simulink model "WindT_Control"  (R2026a)
settings: Solver=VariableStepAuto  StopTime=t(end)
InitFcn:
  | wtModelFile = get_param(bdroot, 'FileName'); wtProjectRoot = fileparts(fileparts(wtModelFile)); wtScriptsDir = fullfile(wtProjectRoot, 'scripts'); addpath(wtScriptsDir); init_wt(get_wind_case(), false);
model workspace (MAT data in the model file):
  surfaceBlockParameters = Simulink.LookupTable
  surfaceBlockParameters.Table = Simulink.lookuptable.Table
  surfaceBlockParameters.Table.Value = [0.000629396007942 0.006627327118 0.0623376026933 0.200719842793 0.356874891063 0.394066762825 0.350958924947 0.335467287882 0.311487736698 0.227563659042 0.0973704524374 0.0013612480249 ... (121 elements, 11x11)]
  surfaceBlockParameters.Table.Dimensions = [11 11]
  surfaceBlockParameters.Table.DataType = 'auto'
  surfaceBlockParameters.Table.FieldName = 'Table_Cp_'
  surfaceBlockParameters.Breakpoints(1) = Simulink.lookuptable.Breakpoint
  surfaceBlockParameters.Breakpoints(1).Value = [0.54 2.14 3.74 5.34 6.94 8.54 10.14 11.74 13.34 14.94 16.54]
  surfaceBlockParameters.Breakpoints(1).TunableSizeName = 'N1'
  surfaceBlockParameters.Breakpoints(1).TunableSizeValue = -1
  surfaceBlockParameters.Breakpoints(1).Dimensions = [1 11]
  surfaceBlockParameters.Breakpoints(1).DataType = 'auto'
  surfaceBlockParameters.Breakpoints(1).FieldName = 'BP1_Lambda'
  surfaceBlockParameters.Breakpoints(2) = Simulink.lookuptable.Breakpoint
  surfaceBlockParameters.Breakpoints(2).Value = [-8 -3.7 0.6 4.9 9.2 13.5 17.8 22.1 26.4 30.7 35]
  surfaceBlockParameters.Breakpoints(2).TunableSizeName = 'N2'
  surfaceBlockParameters.Breakpoints(2).TunableSizeValue = -1
  surfaceBlockParameters.Breakpoints(2).Dimensions = [1 11]
  surfaceBlockParameters.Breakpoints(2).DataType = 'auto'
  surfaceBlockParameters.Breakpoints(2).FieldName = 'BP2_Beta'
  surfaceBlockParameters.AllowMultipleInstancesOfTypeToHaveDifferentTableBreakpointSizes = 0
  surfaceBlockParameters.SupportTunableSize = 0
  surfaceBlockParameters.StructTypeInfo = Simulink.lookuptable.StructTypeInfo
  surfaceBlockParameters.StructTypeInfo.Name = 'surfaceBlockParameters_type'
  surfaceBlockParameters.StructTypeInfo.DataScope = 'Auto'
undefined symbols (not defined in the file): Beta_ott, C_rated, GBEff, GBRatio, GenEff, Jeq, Kreg2, Omega_0, Omega_ott_high, Omega_ott_low, R, rho
settings Model: Creator=39388  LastModifiedBy=notes

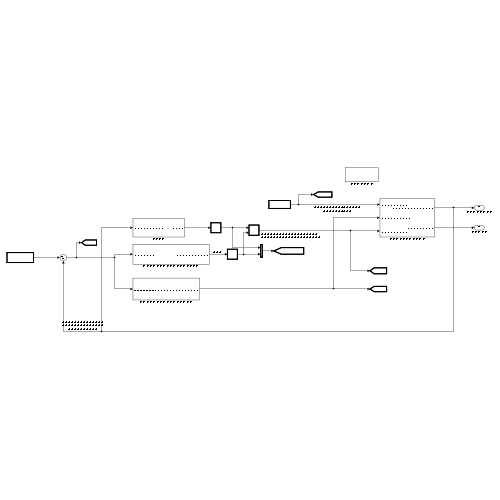
[thumbnail: Simulink's stored preview of the top-level diagram]
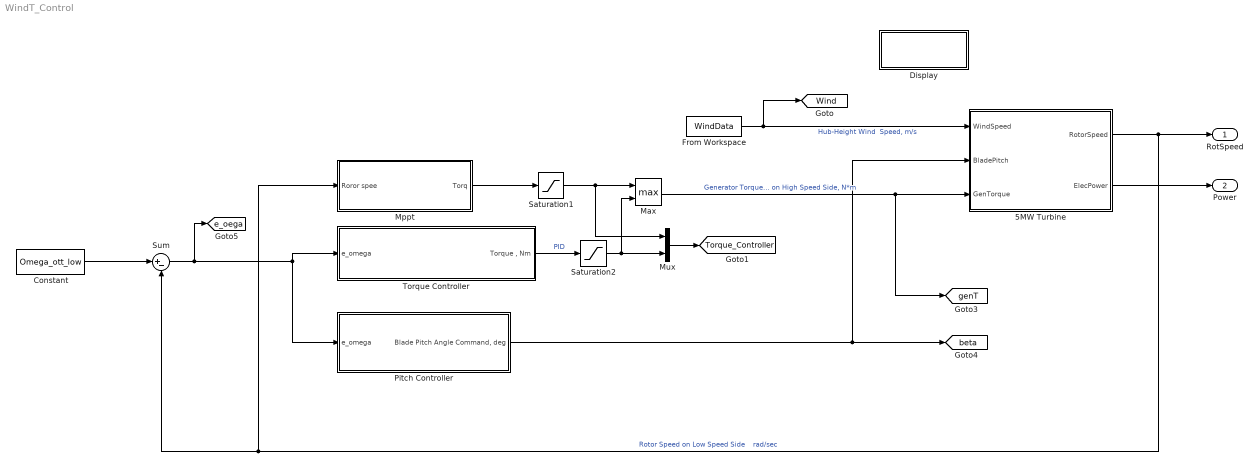
== system WindT_Control ==
  5MW Turbine : Subsystem
  Constant : Constant  Value=Omega_ott_low
  Display : Subsystem
  From Workspace : FromWorkspace  VariableName=WindData
  Max : MinMax  Function=max  Inputs=2
  Mppt : Subsystem
  Mux : Mux  Inputs=2
  Pitch Controller : Subsystem
  Saturation1 : Saturate  UpperLimit=Omega_ott_high^2*Kreg2  LowerLimit=0
  Saturation2 : Saturate  UpperLimit=C_rated/GBRatio  LowerLimit=0
  Sum : Sum  Inputs=|+-
  Torque Controller : Subsystem
  RotSpeed : Outport
  Power : Outport  Port=2
  tag scope: Torque_Controller=global, Wind=global, beta=global, e_oega=global, genT=global
  wires:
  5MW Turbine/2(ElecPower) -> Power/1
  From Workspace/1 -> [Wind], 5MW Turbine/1(WindSpeed)  "Hub-Height Wind  Speed, m/s"
  Pitch Controller/1("Blade Pitch Angle Command, deg") -> [beta], 5MW Turbine/2(BladePitch)
  Mux/1 -> [Torque_Controller]
  Constant/1 -> Sum/1
  Max/1 -> 5MW Turbine/3(GenTorque), [genT]  "Generator Torque on High Speed Side, N*m"
  Torque Controller/1("Torque , Nm") -> Saturation2/1  "PID"
  Mppt/1(Torq) -> Saturation1/1
  5MW Turbine/1("RotorSpeed ") -> RotSpeed/1, Mppt/1(Roror spee), Sum/2  "Rotor Speed on Low Speed Side    rad/sec"
  Sum/1 -> [e_oega], Torque Controller/1(e_omega), Pitch Controller/1(e_omega)
  Saturation1/1 -> Mux/1, Max/1
  Saturation2/1 -> Mux/2, Max/2

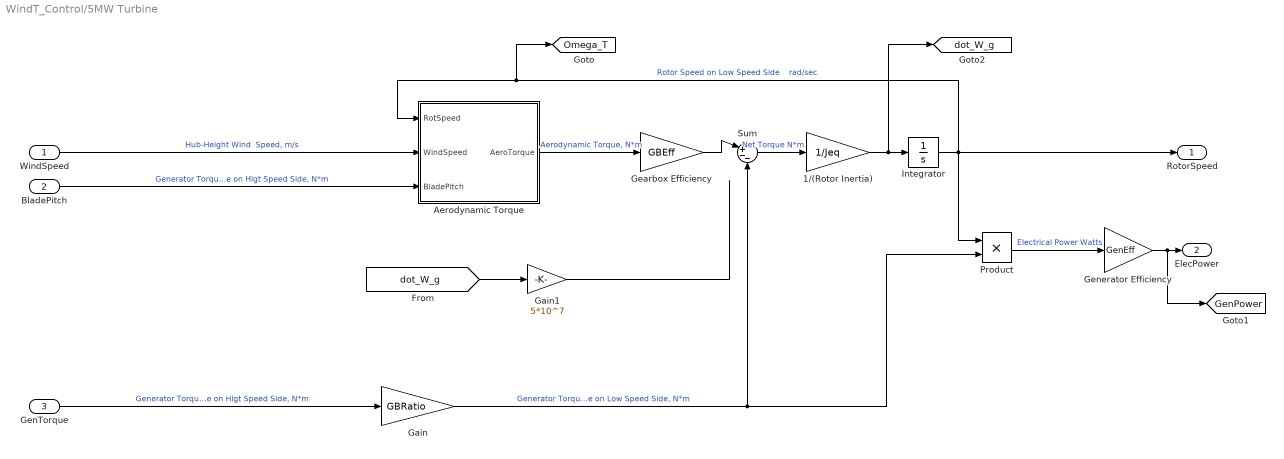
== system WindT_Control/5MW Turbine ==
  WindSpeed : Inport
  BladePitch : Inport  Port=2
  GenTorque : Inport  Port=3
  1/(Rotor Inertia) : Gain  Gain=1/Jeq
  Aerodynamic Torque : Subsystem
  Gain : Gain  Gain=GBRatio
  Gain1 : Gain  Gain=5*10^7
  Gearbox Efficiency : Gain  Gain=GBEff
  Generator Efficiency : Gain  Gain=GenEff
  Integrator : Integrator  InitialCondition=Omega_0
  Product : Product  Inputs=**
  Sum : Sum  Inputs=|+--
  "RotorSpeed " : Outport
  ElecPower : Outport  Port=2
  tag scope: GenPower=global, Omega_T=global, dot_W_g=global
  wires:
  Integrator/1 -> "RotorSpeed "/1, Product/1, [Omega_T], Aerodynamic Torque/1("RotSpeed ")  "Rotor Speed on Low Speed Side    rad/sec"
  Sum/1 -> 1/(Rotor Inertia)/1  "Net Torque N*m"
  Gearbox Efficiency/1 -> Sum/1
  Gain/1 -> Product/2, Sum/3  "Generator Torque on Low Speed Side, N*m"
  1/(Rotor Inertia)/1 -> [dot_W_g], Integrator/1
  WindSpeed/1 -> Aerodynamic Torque/2(WindSpeed)  "Hub-Height Wind  Speed, m/s"
  Aerodynamic Torque/1(AeroTorque) -> Gearbox Efficiency/1  "Aerodynamic Torque, N*m"
  Product/1 -> Generator Efficiency/1  "Electrical Power Watts"
  Generator Efficiency/1 -> [GenPower], ElecPower/1
  BladePitch/1 -> Aerodynamic Torque/3(BladePitch)  "Generator Torque on Higt Speed Side, N*m"
  GenTorque/1 -> Gain/1  "Generator Torque on Higt Speed Side, N*m"
  [dot_W_g] -> Gain1/1
  Gain1/1 -> ?

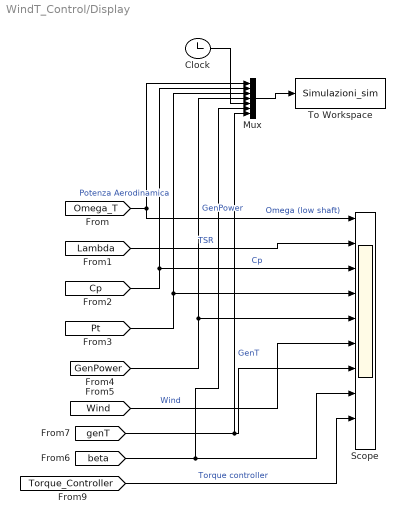
== system WindT_Control/Display ==
  Clock : Clock
  Mux : Mux  Inputs=7
  Scope : Scope  NumInputPorts=10
      settings: ActiveDisplayYMinimum=1.05767  ActiveDisplayYMaximum=1.34149
  To Workspace : ToWorkspace  VariableName=Simulazioni_sim  SampleTime=-1
  wires:
  [Omega_T] -> Mux/1, Scope/1  "Omega (low shaft)"
  [Pt] -> Mux/3, Scope/4  "Potenza Aerodinamica"
  [Lambda] -> Scope/2  "TSR"
  [Cp] -> Mux/2, Scope/3  "Cp"
  [GenPower] -> Mux/4, Scope/5  "GenPower"
  [Wind] -> Scope/6  "Wind"
  Mux/1 -> To Workspace/1
  Clock/1 -> Mux/5
  [beta] -> Mux/6, Scope/8
  [genT] -> Mux/7, Scope/7  "GenT"
  [Torque_Controller] -> Scope/9  "Torque controller"

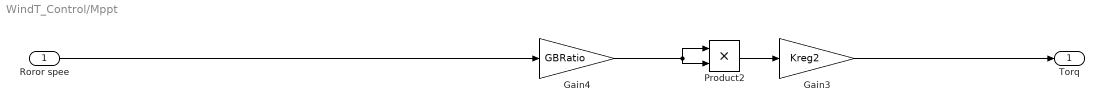
== system WindT_Control/Mppt ==
  Roror spee : Inport
  Gain3 : Gain  Gain=Kreg2
  Gain4 : Gain  Gain=GBRatio
  Product2 : Product
  Torq : Outport
  wires:
  Gain4/1 -> Product2/1, Product2/2
  Gain3/1 -> Torq/1
  Roror spee/1 -> Gain4/1
  Product2/1 -> Gain3/1

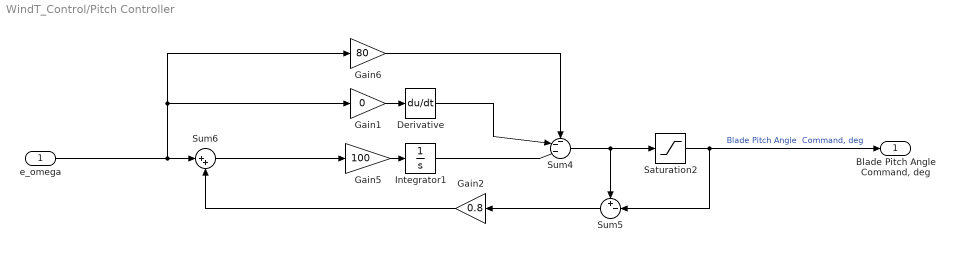
== system WindT_Control/Pitch Controller ==
  e_omega : Inport
  Derivative : Derivative
  Gain1 : Gain  Gain=0
  Gain2 : Gain  Gain=0.8
  Gain5 : Gain  Gain=100
  Gain6 : Gain  Gain=80
  Integrator1 : Integrator
  Saturation2 : Saturate  UpperLimit=90  LowerLimit=Beta_ott
  Sum4 : Sum  Inputs=---|
  Sum5 : Sum  Inputs=+-|
  Sum6 : Sum  Inputs=|++
  "Blade Pitch Angle Command, deg" : Outport
  wires:
  Sum4/1 -> Saturation2/1, Sum5/1
  Gain2/1 -> Sum6/2
  Integrator1/1 -> Sum4/3
  e_omega/1 -> Gain6/1, Gain1/1, Sum6/1
  Sum5/1 -> Gain2/1
  Gain1/1 -> Derivative/1
  Saturation2/1 -> "Blade Pitch Angle Command, deg"/1, Sum5/2  "Blade Pitch Angle  Command, deg"
  Gain6/1 -> Sum4/1
  Gain5/1 -> Integrator1/1
  Derivative/1 -> Sum4/2
  Sum6/1 -> Gain5/1

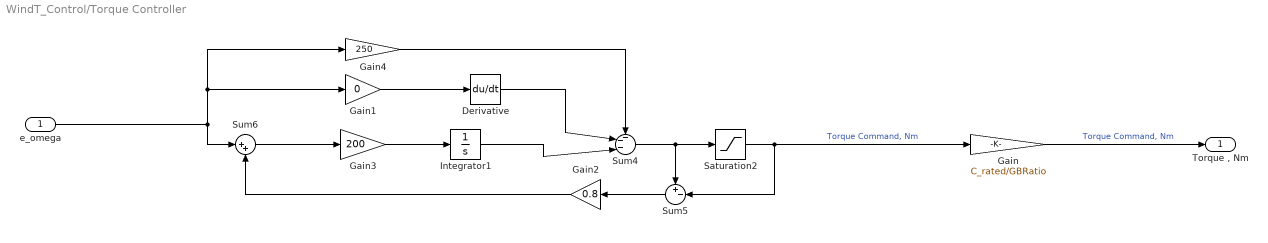
== system WindT_Control/Torque Controller ==
  e_omega : Inport
  Derivative : Derivative
  Gain : Gain  Gain=C_rated/GBRatio
  Gain1 : Gain  Gain=0
  Gain2 : Gain  Gain=0.8
  Gain3 : Gain  Gain=200
  Gain4 : Gain  Gain=250
  Integrator1 : Integrator
  Saturation2 : Saturate  UpperLimit=C_rated/GBRatio  LowerLimit=0
  Sum4 : Sum  Inputs=---|
  Sum5 : Sum  Inputs=+-|
  Sum6 : Sum  Inputs=|++
  "Torque , Nm" : Outport
  wires:
  Gain/1 -> "Torque , Nm"/1  "Torque Command, Nm"
  Gain3/1 -> Integrator1/1
  Sum4/1 -> Saturation2/1, Sum5/1
  Derivative/1 -> Sum4/2
  Gain2/1 -> Sum6/2
  e_omega/1 -> Sum6/1, Gain4/1, Gain1/1
  Saturation2/1 -> Sum5/2, Gain/1  "Torque Command, Nm"
  Gain1/1 -> Derivative/1
  Integrator1/1 -> Sum4/3
  Sum6/1 -> Gain3/1
  Sum5/1 -> Gain2/1
  Gain4/1 -> Sum4/1

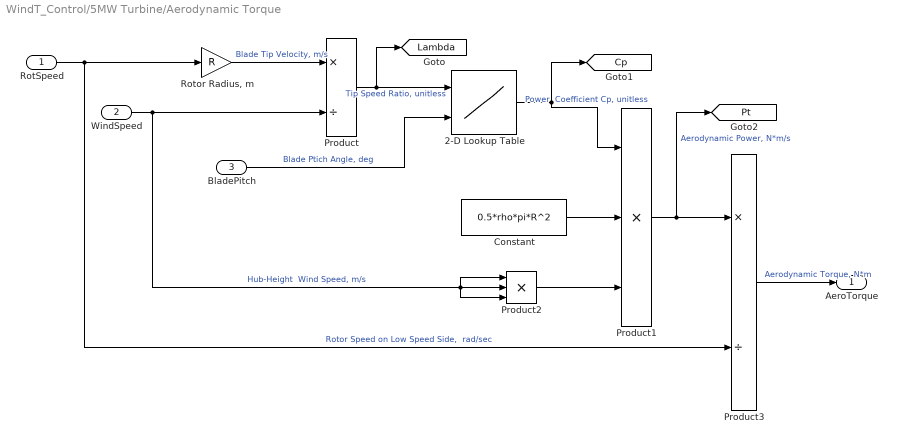
== system WindT_Control/5MW Turbine/Aerodynamic Torque ==
  "RotSpeed " : Inport
  WindSpeed : Inport  Port=2
  BladePitch : Inport  Port=3
  2-D Lookup Table : Lookup_n-D  DataSpecification=Lookup table object  LookupTableObject=surfaceBlockParameters  BreakpointsForDimension1=[1:3]  BreakpointsForDimension2=[1:3]  InternalRulePriority=Speed  RndMeth=Simplest
      settings: InputPortMap=u0,u1
  Constant : Constant  Value=0.5*rho*pi*R^2
  Product : Product  Inputs=*/
  Product1 : Product  Inputs=***
  Product2 : Product  Inputs=***
  Product3 : Product  Inputs=*/
  "Rotor Radius, m" : Gain  Gain=R
  AeroTorque : Outport
  tag scope: Cp=global, Lambda=global, Pt=global
  wires:
  "RotSpeed "/1 -> Product3/2, "Rotor Radius, m"/1  "Rotor Speed on Low Speed Side,  rad/sec"
  "Rotor Radius, m"/1 -> Product/1  "Blade Tip Velocity, m/s"
  WindSpeed/1 -> Product2/3, Product2/1, Product2/2, Product/2  "Hub-Height  Wind Speed, m/s"
  Product/1 -> 2-D Lookup Table/1, [Lambda]  "Tip Speed Ratio, unitless"
  BladePitch/1 -> 2-D Lookup Table/2  "Blade Ptich Angle, deg"
  2-D Lookup Table/1 -> Product1/1, [Cp]  "Power  Coefficient Cp, unitless"
  Constant/1 -> Product1/2
  Product2/1 -> Product1/3
  Product1/1 -> [Pt], Product3/1  "Aerodynamic Power, N*m/s"
  Product3/1 -> AeroTorque/1  "Aerodynamic Torque, N*m"
